simulink model "PedalMapping_26_05"  (Simulink 8.5)
settings: Solver=ode45  StartTime=0.0  StopTime=10.0  RelTol=1e-3
values from neighbouring files (symbols this model uses):
  coast_domain = 0.1    [parameterfile_PedalMapping.m]
  max_coast_Nm = 0    [parameterfile_PedalMapping.m]
  max_torque_Nm = 40    [parameterfile_PedalMapping.m]
  ped_max_limiet = 1    [parameterfile_PedalMapping.m]
  pedal_position_maxacc = 0.9    [parameterfile_PedalMapping.m]
  regen_activation_kph = 15    [parameterfile_PedalMapping.m]
  slewbreak_domain = 0.15    [parameterfile_PedalMapping.m]
  T_min_Nm = -15    [parameterfile_PedalMapping.m]
settings Model: Creator=Sven-VDR  LastModifiedBy=Sven-VDR  CovModelRefEnable=off
settings DataIOCC: SaveFormat=Dataset  SignalLoggingSaveFormat=Dataset
settings OptimizationCC: ExpressionDepthLimit=128
settings DebuggingCC: UnderspecifiedInitializationDetection=Simplified  MergeDetectMultiDrivingBlocksExec=error  FcnCallInpInsideContextMsg=EnableAllAsError  StateNameClashWarn=none
settings HardwareCC: ProdBitPerPointer=64  ProdLargestAtomicFloat=Float  ProdIntDivRoundTo=Zero  ProdEndianess=LittleEndian  ProdHWDeviceType=Specified
settings GRTTargetCC: GeneratePreprocessorConditionals=Use local settings  CombineOutputUpdateFcns=on  GRTInterface=off

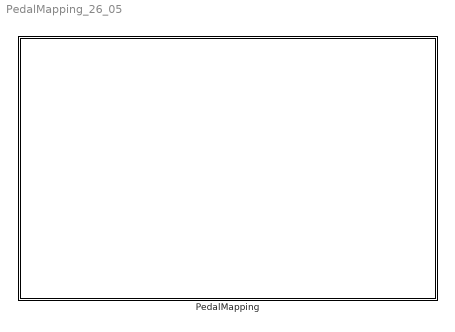
== system PedalMapping_26_05 ==
  PedalMapping : Subsystem

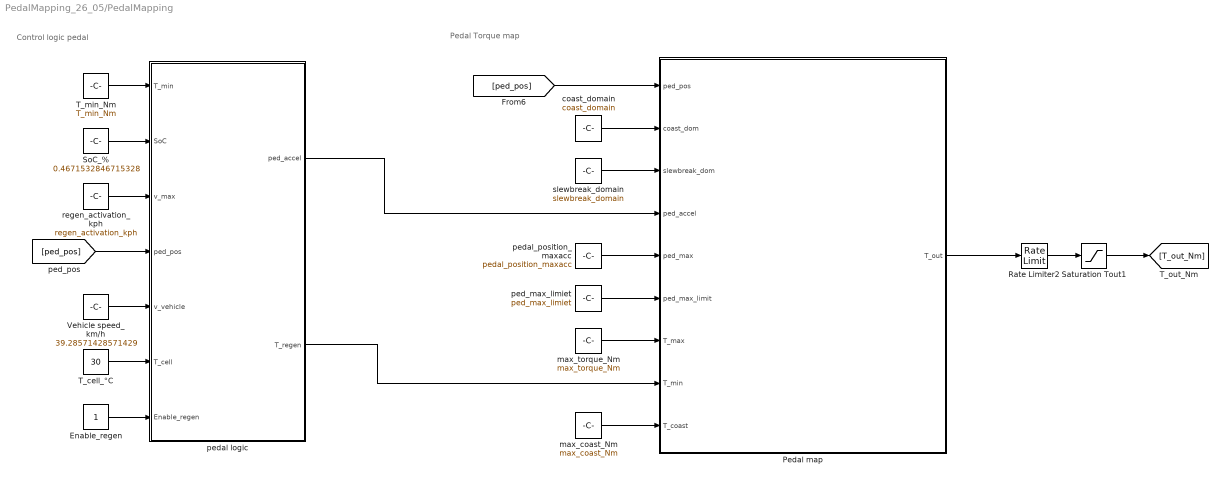
== system PedalMapping_26_05/PedalMapping ==
  note: Pedal Torque map
  note: Control logic pedal
  Enable_regen : Constant
  Pedal map : MATLAB Function  TreatAsAtomicUnit=on
      settings: PermitHierarchicalResolution=ParametersOnly
  Rate Limiter2 : RateLimiter  RisingSlewLimit=2000  FallingSlewLimit=-2000  SampleTimeMode=inherited
  Saturation Tout1 : Saturate  UpperLimit=40  LowerLimit=-40
  SoC_% : Constant  Value=0.4671532846715328
  T_cell_°C : Constant  Value=30
  T_min_Nm : Constant  Value=T_min_Nm
  Vehicle speed_km/h : Constant  Value=39.28571428571429
  coast_domain : Constant  Value=coast_domain
  max_coast_Nm : Constant  Value=max_coast_Nm
  max_torque_Nm : Constant  Value=max_torque_Nm
  ped_max_limiet : Constant  Value=ped_max_limiet
  pedal logic : Stateflow chart  TreatAsAtomicUnit=on
      settings: PermitHierarchicalResolution=ParametersOnly
  pedal_position_maxacc : Constant  Value=pedal_position_maxacc
  regen_activation_kph : Constant  Value=regen_activation_kph
  slewbreak_domain : Constant  Value=slewbreak_domain
  wires:
  Vehicle speed_km/h/1 -> pedal logic/5(v_vehicle)
  Rate Limiter2/1 -> Saturation Tout1/1
  coast_domain/1 -> Pedal map/2(coast_dom)
  T_min_Nm/1 -> pedal logic/1(T_min)
  pedal_position_maxacc/1 -> Pedal map/5(ped_max)
  slewbreak_domain/1 -> Pedal map/3(slewbreak_dom)
  Saturation Tout1/1 -> [T_out_Nm]
  [ped_pos] -> Pedal map/1(ped_pos)
  T_cell_°C/1 -> pedal logic/6(T_cell)
  SoC_%/1 -> pedal logic/2(SoC)
  ped_max_limiet/1 -> Pedal map/6(ped_max_limit)
  pedal logic/2(T_regen) -> Pedal map/8(T_min)
  max_coast_Nm/1 -> Pedal map/9(T_coast)
  regen_activation_kph/1 -> pedal logic/3(v_max)
  Enable_regen/1 -> pedal logic/7(Enable_regen)
  pedal logic/1(ped_accel) -> Pedal map/4(ped_accel)
  [ped_pos] -> pedal logic/4(ped_pos)
  max_torque_Nm/1 -> Pedal map/7(T_max)
  Pedal map/1(T_out) -> Rate Limiter2/1

== matlab function PedalMapping/Pedal map ==
  data: ped_pos input double; coast_dom input double; T_out output double; slewbreak_dom input double; ped_accel input double; ped_max input double; ped_max_limit input double; T_max input double; T_min input double; T_coast input double
function T_out = Pedalmap_eq(ped_pos,coast_dom,slewbreak_dom,ped_accel,ped_max,ped_max_limit,T_max,T_min,T_coast)
%%Accelerator pedal mapping:

ped_regen=ped_accel-coast_dom; %pedal postion - start regen - variable in function of velocity
ped_zero=ped_regen-slewbreak_dom; %pedal postion - start max regen - variable in function of velocity

slewrate_acc=(T_max-T_coast)/(ped_max-ped_accel); %slewrate acceleration region
slewrate_regen=(T_min-T_coast)/(ped_zero-ped_regen);%slewrate regen region

% acceleration pedal map eq.
T_out=T_min*(heavi(ped_pos,-0.1)-heavi(ped_pos,ped_zero)) + (slewrate_regen*(ped_pos-ped_regen)+T_coast)*(heavi(ped_pos,ped_zero)-heavi(ped_pos,ped_regen))+T_coast*(heavi(ped_pos,ped_regen)-heavi(ped_pos,ped_accel))+(slewrate_acc*(ped_pos-ped_accel)+T_coast)*(heavi(ped_pos,ped_accel)-heavi(ped_pos,ped_max))+T_max*(heavi(ped_pos,ped_max-heavi(ped_pos,ped_max_limit)));

== stateflow chart PedalMapping/pedal logic ==
  state Driving
    state Disable_regen
      entry:
      ped_accel=0.45;
      T_regen=0;
    state Activate_regen
      entry:
      ped_accel=0.45;
      T0= -5; %Regentorque at v_lim [Nm]
      during:
      % velocity dependant braking torque
      if v_vehicle<15
      T_regen=T_min/(15-5)*(v_vehicle-5);
      elseif v_vehicle<50
      T_regen=T_min;
      else
      T_regen=max((T_min-T0)/(50-100)*(v_vehicle-100)+T0,0);
      end
    (default) -> Disable_regen
    Disable_regen -> Activate_regen : [SoC<0.95 && Enable_regen==1]
    Activate_regen -> Disable_regen : [SoC>0.95 || T_cell>55 || Enable_regen==0]
  state Standstill
    entry:
    T_regen=0;
    ped_accel=0.1; %
    during:
    %velocity dependent coasting until v_max
    if ped_pos>0.1
    ped_accel=min(ped_pos* (v_vehicle/v_max),0.45); %Offset of 0.1
    end
    exit:
    ped_accel=0.45;
  (default) -> Standstill
  Driving -> Standstill : [v_vehicle<=5]
  Standstill -> Driving : [v_vehicle >v_max&&ped_pos>0.45]
  data: T_min input double; SoC input double; v_max input double; ped_pos input double; v_vehicle input double; ped_accel output double; T_regen output double; T0 local double; T_cell input double; Enable_regen input double
